simulink model "HomeTaskModel"  (R2022b)
settings: Solver=VariableStepAuto  StartTime=0.0  StopTime=1  RelTol=1e-3
undefined symbols (not defined in the file): alpha_filt, x0
settings Model: Creator=ilya  LastModifiedBy=ilya

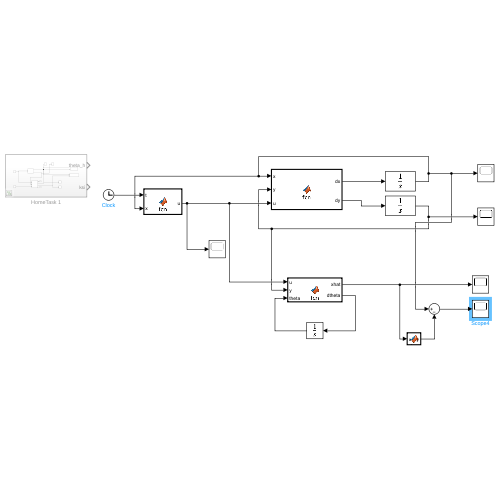
[thumbnail: Simulink's stored preview of the top-level diagram]
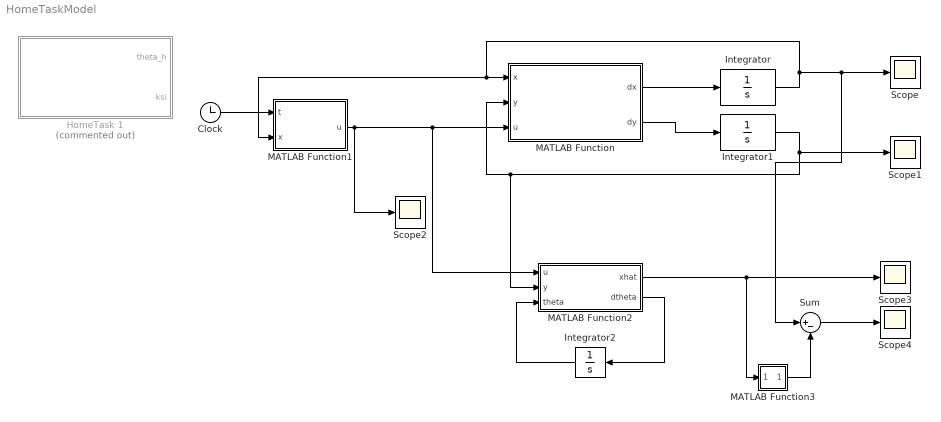
== system HomeTaskModel ==
  Clock : Clock
  HomeTask 1 : Subsystem  Commented=on
  Integrator : Integrator  InitialCondition=[0.5 -1]
  Integrator1 : Integrator  InitialCondition=[10 -12]
  Integrator2 : Integrator  InitialCondition=[0;0]
  MATLAB Function : MATLAB Function  TreatAsAtomicUnit=on
  MATLAB Function1 : MATLAB Function  TreatAsAtomicUnit=on
  MATLAB Function2 : MATLAB Function  TreatAsAtomicUnit=on
  MATLAB Function3 : MATLAB Function  TreatAsAtomicUnit=on
  Scope{,1..4} (5 alike) : Scope
  Sum : Sum  Inputs=|+-
  wires:
  MATLAB Function/1(dx) -> Integrator/1
  MATLAB Function/2(dy) -> Integrator1/1
  Integrator/1 -> MATLAB Function1/2(x), MATLAB Function/1(x), Sum/1, Scope/1
  Integrator1/1 -> Scope1/1, MATLAB Function2/2(y), MATLAB Function/2(y)
  MATLAB Function1/1(u) -> Scope2/1, MATLAB Function2/1(u), MATLAB Function/3(u)
  Clock/1 -> MATLAB Function1/1(t)
  MATLAB Function2/2(dtheta) -> Integrator2/1
  MATLAB Function2/1(xhat) -> MATLAB Function3/1(u), Scope3/1
  Sum/1 -> Scope4/1
  Integrator2/1 -> MATLAB Function2/3(theta)
  MATLAB Function3/1(y) -> Sum/2

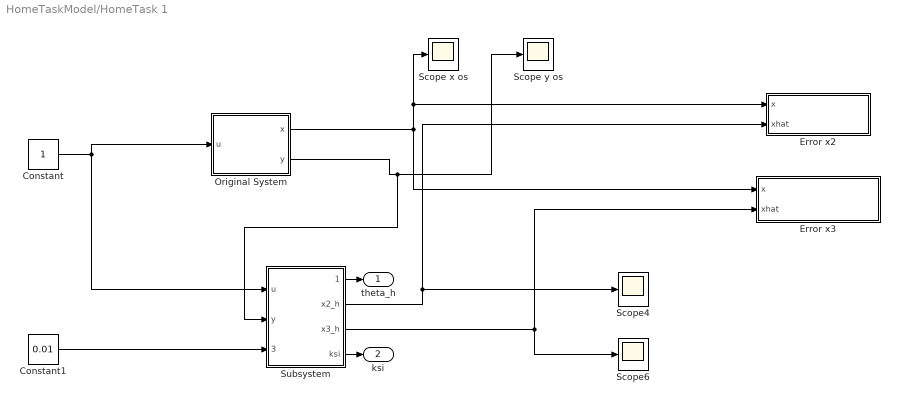
== system HomeTaskModel/HomeTask 1 ==
  Constant : Constant
  Constant1 : Constant  Value=0.01
  Error x2 : Subsystem
  Error x3 : Subsystem
  Original System : Subsystem
  Scope x os : Scope
  Scope y os : Scope
  Scope4 : Scope
  Scope6 : Scope
  Subsystem : Subsystem
  theta_h : Outport
  ksi : Outport  Port=2
  wires:
  Original System/2(y) -> Subsystem/2(y), Scope y os/1
  Subsystem/3(x3_h) -> Scope6/1, Error x3/2(xhat)
  Constant/1 -> Original System/1(u), Subsystem/1(u)
  Subsystem/2(x2_h) -> Scope4/1, Error x2/2(xhat)
  Original System/1(x) -> Error x2/1(x), Scope x os/1, Error x3/1(x)
  Subsystem/4(ksi) -> ksi/1
  Constant1/1 -> Subsystem/3(gamma)
  Subsystem/1(theta_h) -> theta_h/1

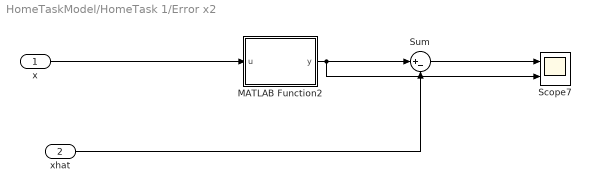
== system HomeTaskModel/HomeTask 1/Error x2 ==
  x : Inport
  xhat : Inport  Port=2
  MATLAB Function2 : MATLAB Function  TreatAsAtomicUnit=on
  Scope7 : Scope  NumInputPorts=2
  Sum : Sum  Inputs=|+-
  wires:
  xhat/1 -> Sum/2
  Sum/1 -> Scope7/1
  MATLAB Function2/1(y) -> Scope7/2, Sum/1
  x/1 -> MATLAB Function2/1(u)

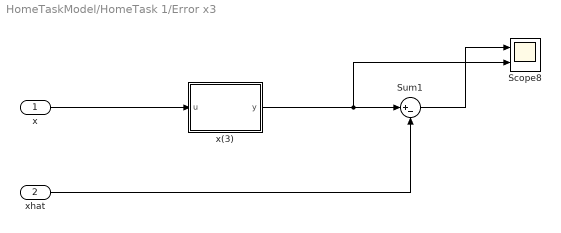
== system HomeTaskModel/HomeTask 1/Error x3 ==
  x : Inport
  xhat : Inport  Port=2
  Scope8 : Scope  NumInputPorts=2
  Sum1 : Sum  Inputs=|+-
  x(3) : MATLAB Function  TreatAsAtomicUnit=on
  wires:
  Sum1/1 -> Scope8/1
  x(3)/1(y) -> Scope8/2, Sum1/1
  xhat/1 -> Sum1/2
  x/1 -> x(3)/1(u)

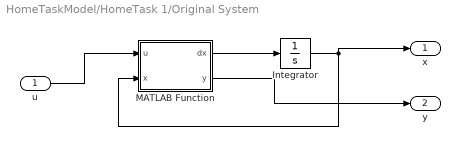
== system HomeTaskModel/HomeTask 1/Original System ==
  u : Inport
  Integrator : Integrator  InitialCondition=x0
  MATLAB Function : MATLAB Function  TreatAsAtomicUnit=on
  x : Outport
  y : Outport  Port=2
  wires:
  MATLAB Function/1(dx) -> Integrator/1
  MATLAB Function/2(y) -> y/1
  u/1 -> MATLAB Function/1(u)
  Integrator/1 -> MATLAB Function/2(x), x/1

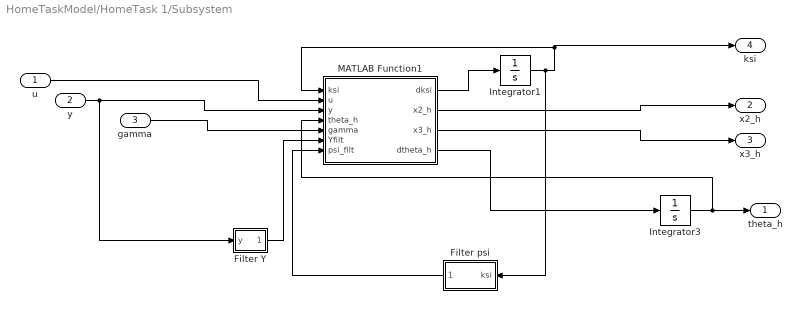
== system HomeTaskModel/HomeTask 1/Subsystem ==
  u : Inport
  y : Inport  Port=2
  gamma : Inport  Port=3
  Filter Y : Subsystem
  Filter psi : Subsystem
  Integrator1 : Integrator  InitialCondition=[0 0]
  Integrator3 : Integrator  InitialCondition=0.01
  MATLAB Function1 : MATLAB Function  TreatAsAtomicUnit=on
  theta_h : Outport
  x2_h : Outport  Port=2
  x3_h : Outport  Port=3
  ksi : Outport  Port=4
  wires:
  u/1 -> MATLAB Function1/2(u)
  MATLAB Function1/3(x3_h) -> x3_h/1
  MATLAB Function1/2(x2_h) -> x2_h/1
  MATLAB Function1/1(dksi) -> Integrator1/1
  Integrator1/1 -> Filter psi/1(ksi), ksi/1, MATLAB Function1/1(ksi)
  y/1 -> Filter Y/1(y), MATLAB Function1/3(y)
  gamma/1 -> MATLAB Function1/5(gamma)
  Integrator3/1 -> MATLAB Function1/4(theta_h), theta_h/1
  MATLAB Function1/4(dtheta_h) -> Integrator3/1
  Filter Y/1(Yfilt) -> MATLAB Function1/6(Yfilt)
  Filter psi/1(psi_filt) -> MATLAB Function1/7(psi_filt)

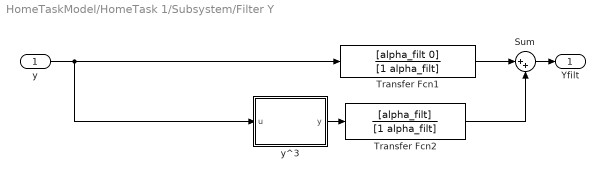
== system HomeTaskModel/HomeTask 1/Subsystem/Filter Y ==
  y : Inport
  Sum : Sum  Inputs=|++
  Transfer Fcn1 : TransferFcn  Numerator=[alpha_filt 0]  Denominator=[1 alpha_filt]
  Transfer Fcn2 : TransferFcn  Numerator=[alpha_filt]  Denominator=[1 alpha_filt]
  y^3 : MATLAB Function  TreatAsAtomicUnit=on
  Yfilt : Outport
  wires:
  y^3/1(y) -> Transfer Fcn2/1
  Transfer Fcn2/1 -> Sum/2
  Transfer Fcn1/1 -> Sum/1
  Sum/1 -> Yfilt/1
  y/1 -> y^3/1(u), Transfer Fcn1/1

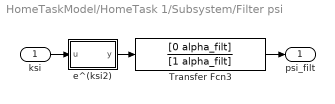
== system HomeTaskModel/HomeTask 1/Subsystem/Filter psi ==
  ksi : Inport
  Transfer Fcn3 : TransferFcn  Numerator=[0 alpha_filt]  Denominator=[1 alpha_filt]
  e^(ksi2) : MATLAB Function  TreatAsAtomicUnit=on
  psi_filt : Outport
  wires:
  e^(ksi2)/1(y) -> Transfer Fcn3/1
  ksi/1 -> e^(ksi2)/1(u)
  Transfer Fcn3/1 -> psi_filt/1

== matlab function HomeTaskModel/MATLAB Function3 ==
  data: u input; y output
function y = fcn(u)

y = [u(1) u(2)];

== matlab function HomeTaskModel/HomeTask 1/Subsystem/MATLAB Function1 ==
  data: ksi input; u input; dksi output; y input; theta_h input; gamma input; x2_h output; x3_h output; Yfilt input; psi_filt input; dtheta_h output
function [dksi,x2_h, x3_h, dtheta_h] = fcn(ksi, u, y, theta_h, gamma, Yfilt, psi_filt)
    dksi1 = -ksi(1) + y^2 + sin(y);
    dksi2 = u*y + (y^2 + 1)^(-1);
    dtheta_h = gamma * psi_filt * (Yfilt - psi_filt * theta_h);
    x2_h = ksi(1);
    x3_h = ksi(2) + real(log(complex(theta_h)));%log(theta_h);
    dksi = [dksi1, dksi2];

== matlab function HomeTaskModel/HomeTask 1/Original System/MATLAB Function ==
  data: dx output; u input; y output; x input
function [dx,y] = fcn(u,x)

dx1 = -x(1)^3 + exp(x(3));
dx2 = -x(2) + x(1)^2 + sin(x(1));
dx3 = 1/(x(1)^2 + 1) + x(1) * u;
y = x(1);
dx = [dx1, dx2, dx3];

== matlab function HomeTaskModel/MATLAB Function ==
  data: x input; y input; u input; dx output; dy output
function [dx, dy] = fcn(x, y, u)
L1 = 10 * 0.001;
L3 = 5 * 0.001;
C2 = 22 * 0.000001;
C4 = 22.9 * 0.000001;
G = 0.0447 ;
E = 12;

dx1 = -(1-u)*y(1) / L1 + E / L1;
dx2 = y(2)/C4 - G*x(2) / C4;
dy1 = (1-u)*x(1)/C2 + u*y(2) / C2;
dy2 = -u*y(1)/L3 - x(2)/L3;
dx = [dx1 dx2];
dy = [dy1 dy2];

== matlab function HomeTaskModel/MATLAB Function1 ==
  data: t input; u output; x input
function u = fcn(t, x)
E = 12;
v2 = 10;
G = 0.0447;
lambda0 = 1;

Vd = 25;
if (t >= 0.2 && t < 0.4)
    Vd = 30;
elseif (t >= 0.4 && t < 0.6)
    Vd = 15;
elseif (t >= 0.6 && t < 0.8)
    Vd = 5;
else
    Vd = 20;
end

lambda = lambda0 * min(abs(Vd)/(abs(Vd) + E), E / (abs(Vd) + E) );
Vd = abs(Vd);
u = abs(Vd)/(abs(Vd) + E) + lambda * (G*Vd*v2 + E*(x(2)-x(1))) / (1 + (G*Vd*v2+E*(x(2)-x(1)))^2);

== matlab function HomeTaskModel/HomeTask 1/Error x2/MATLAB Function2 ==
  data: u input; y output
function y = fcn(u)

y = u(2);

== matlab function HomeTaskModel/HomeTask 1/Error x3/x(3) ==
  data: u input; y output
function y = fcn(u)

y = u(3);

== matlab function HomeTaskModel/HomeTask 1/Subsystem/Filter Y/y^3 ==
  data: u input; y output
function y = fcn(u)

y = u^3;

== matlab function HomeTaskModel/HomeTask 1/Subsystem/Filter psi/e^(ksi2) ==
  data: u input; y output
function y = fcn(u)

y = exp(u(2));

== matlab function HomeTaskModel/MATLAB Function2 ==
  data: u input; xhat output; y input; theta input; dtheta output
function [xhat, dtheta] = fcn(u, y, theta)
L1 = 10 * 0.001;
L3 = 5 * 0.001;
C2 = 22 * 0.000001;
C4 = 22.9 * 0.000001;
G = 0.0447 ;
E = 12;

gamma1 = 50; gamma2 = 1;

%dtheta1 = -gamma1*(1-u)*(theta(1) + C2*gamma1*y(1)) + gamma1*u*y(2) + (E-(1-u)*y(1))/L1;
dtheta1 = (E - (1-u)*y(1))/L1 - gamma1*((1-u)*(theta(1)+C2*gamma1*y(1)) + u*y(2));
dtheta2 = (y(2) - G*(theta(2)-L3*gamma2*y(2)))/C4 - gamma(2)*(u*y(1) + theta(2) - L3*gamma2*y(2));

xhat = theta + [C2*gamma1*y(1); L3*gamma2*y(2)];
dtheta = [dtheta1; dtheta2];
